simulink model "MTotalRequested"  (R2024b)
settings: configuration reference "STM32H7_Config" (kept outside this file)
undefined symbols (not defined in the file): PPowerControllerActivation
libraries: simulink x4
settings Model: DataDictionary=Master_Dictionary.sldd  EnableAccessToBaseWorkspace=off  Creator=torni  LastModifiedBy=William
settings ConfigSetRef: SourceName=STM32H7_Config

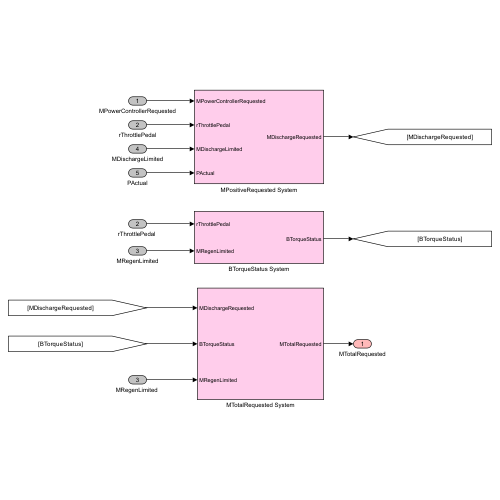
[thumbnail: Simulink's stored preview of the top-level diagram]
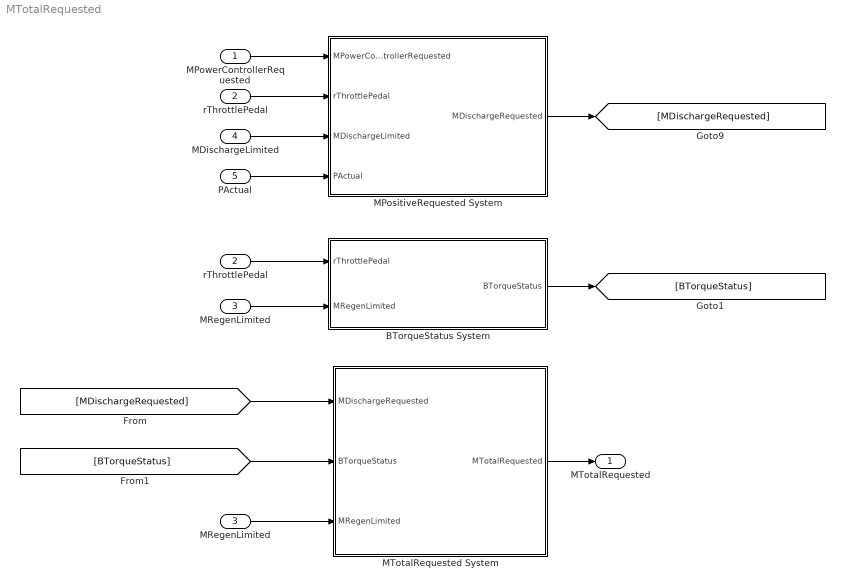
== system MTotalRequested ==
  MPowerControllerRequested : Inport  OutDataTypeStr=double
  rThrottlePedal : Inport  Port=2  OutDataTypeStr=double
  MRegenLimited : Inport  Port=3  OutDataTypeStr=double
  MDischargeLimited : Inport  Port=4  OutDataTypeStr=double
  PActual : Inport  Port=5  OutDataTypeStr=double
  BTorqueStatus System : Subsystem
  MPositiveRequested System : Subsystem
  "MRegenLimited " : InportShadow  Port=3  OutDataTypeStr=double
  MTotalRequested System : Subsystem
  "rThrottlePedal " : InportShadow  Port=2  OutDataTypeStr=double
  MTotalRequested : Outport  OutDataTypeStr=double  VectorParamsAs1DForOutWhenUnconnected=off
  wires:
  rThrottlePedal/1 -> MPositiveRequested System/2(rThrottlePedal)
  PActual/1 -> MPositiveRequested System/4(PActual)
  MDischargeLimited/1 -> MPositiveRequested System/3(MDischargeLimited)
  MPowerControllerRequested/1 -> MPositiveRequested System/1(MPowerControllerRequested)
  MPositiveRequested System/1(MDischargeRequested) -> [MDischargeRequested]
  BTorqueStatus System/1(BTorqueStatus) -> [BTorqueStatus]
  "rThrottlePedal "/1 -> BTorqueStatus System/1(rThrottlePedal)
  MRegenLimited/1 -> BTorqueStatus System/2(MRegenLimited)
  [MDischargeRequested] -> MTotalRequested System/1(MDischargeRequested)
  [BTorqueStatus] -> MTotalRequested System/2(BTorqueStatus)
  "MRegenLimited "/1 -> MTotalRequested System/3(MRegenLimited)
  MTotalRequested System/1(MTotalRequested) -> MTotalRequested/1

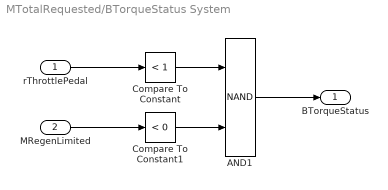
== system MTotalRequested/BTorqueStatus System ==
  rThrottlePedal : Inport  OutDataTypeStr=double
  MRegenLimited : Inport  Port=2  OutDataTypeStr=double
  AND1 : Logic  Operator=NAND  AllPortsSameDT=off  OutDataTypeStr=boolean
  Compare To Constant : simulink/Logic and Bit Operations/Compare To Constant  relop=<  const=1  OutDataTypeStr=boolean
  Compare To Constant1 : simulink/Logic and Bit Operations/Compare To Constant  relop=<  const=0  OutDataTypeStr=boolean
  BTorqueStatus : Outport  OutDataTypeStr=boolean  VectorParamsAs1DForOutWhenUnconnected=off
  wires:
  AND1/1 -> BTorqueStatus/1
  Compare To Constant/1 -> AND1/1
  Compare To Constant1/1 -> AND1/2
  rThrottlePedal/1 -> Compare To Constant/1
  MRegenLimited/1 -> Compare To Constant1/1

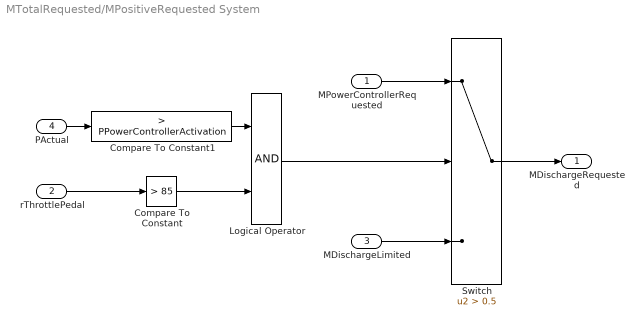
== system MTotalRequested/MPositiveRequested System ==
  MPowerControllerRequested : Inport  OutDataTypeStr=double
  rThrottlePedal : Inport  Port=2  OutDataTypeStr=double
  MDischargeLimited : Inport  Port=3  OutDataTypeStr=double
  PActual : Inport  Port=4  OutDataTypeStr=double
  Compare To Constant : simulink/Logic and Bit Operations/Compare To Constant  relop=>  const=85  OutDataTypeStr=boolean
  Compare To Constant1 : simulink/Logic and Bit Operations/Compare To Constant  relop=>  const=PPowerControllerActivation  OutDataTypeStr=boolean
  Logical Operator : Logic  AllPortsSameDT=off  OutDataTypeStr=boolean
  Switch : Switch  Criteria=u2 > Threshold  Threshold=0.5  SaturateOnIntegerOverflow=off  InputSameDT=off
  MDischargeRequested : Outport  OutDataTypeStr=double  VectorParamsAs1DForOutWhenUnconnected=off
  wires:
  Switch/1 -> MDischargeRequested/1
  Compare To Constant1/1 -> Logical Operator/1
  MDischargeLimited/1 -> Switch/3
  Compare To Constant/1 -> Logical Operator/2
  rThrottlePedal/1 -> Compare To Constant/1
  MPowerControllerRequested/1 -> Switch/1
  Logical Operator/1 -> Switch/2
  PActual/1 -> Compare To Constant1/1

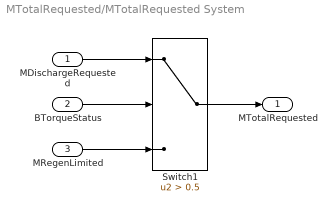
== system MTotalRequested/MTotalRequested System ==
  MDischargeRequested : Inport  OutDataTypeStr=double
  BTorqueStatus : Inport  Port=2  OutDataTypeStr=boolean
  MRegenLimited : Inport  Port=3  OutDataTypeStr=double
  Switch1 : Switch  Criteria=u2 > Threshold  Threshold=0.5  SaturateOnIntegerOverflow=off  InputSameDT=off
  MTotalRequested : Outport  OutDataTypeStr=double  VectorParamsAs1DForOutWhenUnconnected=off
  wires:
  Switch1/1 -> MTotalRequested/1
  MDischargeRequested/1 -> Switch1/1
  BTorqueStatus/1 -> Switch1/2
  MRegenLimited/1 -> Switch1/3
